simulink model "Metodo_Alfaro_IAE"  (R2021a)
settings: Solver=VariableStepAuto  StartTime=0.0  StopTime=100  RelTol=1e-3
settings Model: Creator=roberto  LastModifiedBy=roberto

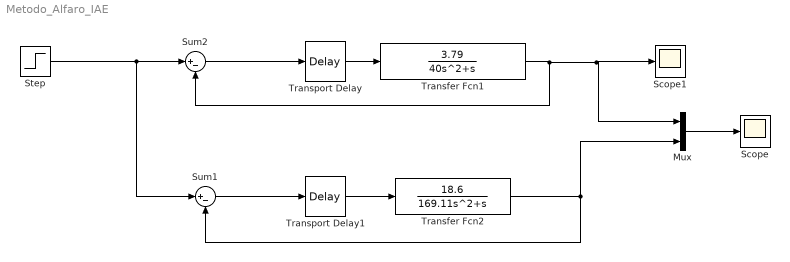
== system Metodo_Alfaro_IAE ==
  Mux : Mux  Inputs=2
  Scope : Scope
  Scope1 : Scope
  Step : Step  SampleTime=0
  Sum1 : Sum  Inputs=|+-
  Sum2 : Sum  Inputs=|+-
  Transfer Fcn1 : TransferFcn  Numerator=[3.79]  Denominator=[40 1 0]
  Transfer Fcn2 : TransferFcn  Numerator=[18.6]  Denominator=[169.11 1 0]
  Transport Delay : TransportDelay  DelayTime=2
  Transport Delay1 : TransportDelay  DelayTime=2
  wires:
  Transfer Fcn2/1 -> Mux/2, Sum1/2
  Sum1/1 -> Transport Delay1/1
  Step/1 -> Sum1/1, Sum2/1
  Transport Delay/1 -> Transfer Fcn1/1
  Sum2/1 -> Transport Delay/1
  Mux/1 -> Scope/1
  Transfer Fcn1/1 -> Scope1/1, Mux/1, Sum2/2
  Transport Delay1/1 -> Transfer Fcn2/1
